simulink model "NotasMusicales"  (R2023a)
settings: Solver=VariableStepAuto  StartTime=0.0  StopTime=5  RelTol=1e-3
values from neighbouring files (symbols this model uses):
  fd = fa / fs    (= 0.029366)    [Frecuencias_musicales.m]
libraries: dspsnks4 x1
settings Model: Creator=carlo  LastModifiedBy=carlo

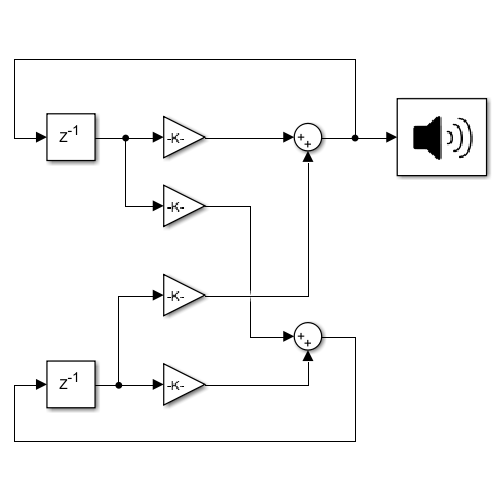
[thumbnail: Simulink's stored preview of the top-level diagram]
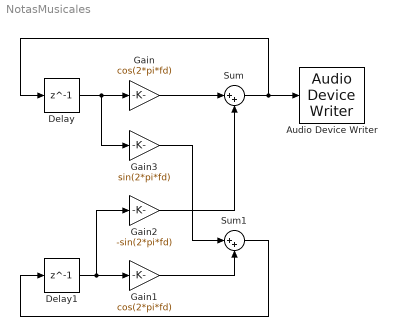
== system NotasMusicales ==
  Audio Device Writer : dspsnks4/Audio Device Writer  Driver=DirectSound  Device=Altavoz/Auricular (Realtek(R) Audio)  InheritSampleRate=on  SampleRate=44100  BitDepth=16-bit integer  BufferSize=4096  NumBuffers=10  DefaultOutputChannelMapping=on  OutputChannelMapping=1:2  OutputNumUnderrunSamples=off  DriverIdx=1  DeviceWarnFlag=''
  Delay : Delay  DelayLength=1  SampleTime=1/10000
  Delay1 : Delay  DelayLength=1  InitialCondition=1  SampleTime=1/10000
  Gain : Gain  Gain=cos(2*pi*fd)
  Gain1 : Gain  Gain=cos(2*pi*fd)
  Gain2 : Gain  Gain=-sin(2*pi*fd)
  Gain3 : Gain  Gain=sin(2*pi*fd)
  Sum : Sum  Inputs=|++
  Sum1 : Sum  Inputs=|++
  wires:
  Delay/1 -> Gain3/1, Gain/1
  Delay1/1 -> Gain2/1, Gain1/1
  Gain/1 -> Sum/1
  Gain2/1 -> Sum/2
  Gain3/1 -> Sum1/1
  Gain1/1 -> Sum1/2
  Sum/1 -> Audio Device Writer/1, Delay/1
  Sum1/1 -> Delay1/1
